simulink model "AutoRS_Blatt_und_Turm"  (R2022b)
settings: Solver=FixedStepAuto  StartTime=0.0  StopTime=50  FixedStep=1e-4  RelTol=1e-3
undefined symbols (not defined in the file): F_s_final
settings Model: Creator=Sebastian  LastModifiedBy=Aaron

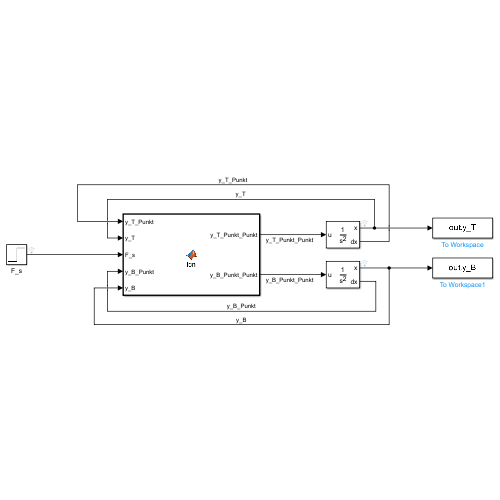
[thumbnail: Simulink's stored preview of the top-level diagram]
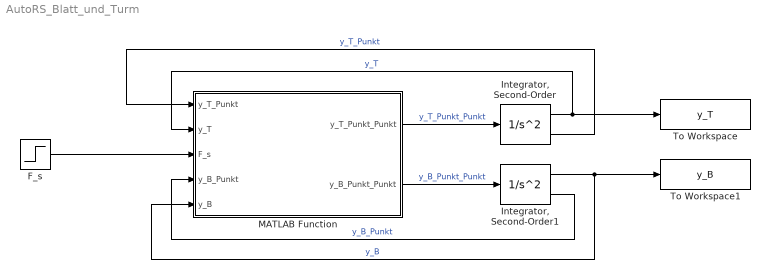
== system AutoRS_Blatt_und_Turm ==
  F_s : Step  Time=0  After=F_s_final  SampleTime=0
  "Integrator, Second-Order" : SecondOrderIntegrator  ICX=0
  "Integrator, Second-Order1" : SecondOrderIntegrator  ICX=0
  MATLAB Function : MATLAB Function  TreatAsAtomicUnit=on
  To Workspace : ToWorkspace  VariableName=y_T  SaveFormat=Timeseries  SampleTime=-1
  To Workspace1 : ToWorkspace  VariableName=y_B  SaveFormat=Timeseries  SampleTime=-1
  wires:
  MATLAB Function/1(y_T_Punkt_Punkt) -> "Integrator, Second-Order"/1  "y_T_Punkt_Punkt"
  "Integrator, Second-Order"/2 -> MATLAB Function/1(y_T_Punkt)  "y_T_Punkt"
  "Integrator, Second-Order"/1 -> To Workspace/1, MATLAB Function/2(y_T)  "y_T"
  MATLAB Function/2(y_B_Punkt_Punkt) -> "Integrator, Second-Order1"/1  "y_B_Punkt_Punkt"
  "Integrator, Second-Order1"/2 -> MATLAB Function/4(y_B_Punkt)  "y_B_Punkt"
  "Integrator, Second-Order1"/1 -> To Workspace1/1, MATLAB Function/5(y_B)  "y_B"
  F_s/1 -> MATLAB Function/3(F_s)

== matlab function AutoRS_Blatt_und_Turm/MATLAB Function ==
  data: y_T_Punkt input; y_T input; F_s input; y_T_Punkt_Punkt output; y_B_Punkt input; y_B input; y_B_Punkt_Punkt output; param_const parameter
function [y_T_Punkt_Punkt, y_B_Punkt_Punkt] = fcn(y_T_Punkt, y_T, F_s, y_B_Punkt, y_B, param_const)
    
    % BERECHNUNG
    y_T_Punkt_Punkt = (-param_const.k_T*y_T-param_const.d_T*y_T_Punkt+3*param_const.k_B*(y_B-y_T)+3*param_const.d_B*(y_B_Punkt-y_T_Punkt))/param_const.m_T;
    
    y_B_Punkt_Punkt = (-3*param_const.k_B*(y_B-y_T)-3*param_const.d_B*(y_B_Punkt-y_T_Punkt)+F_s)/(3*param_const.m_B);

end
